simulink model "ACC_model"  (R2021a)
settings: Solver=VariableStepAuto  StartTime=0.0  StopTime=300  RelTol=1e-3
model workspace (MAT data in the model file):
  d0 = 0
undefined symbols (not defined in the file): sigbuilder_block
libraries: simulink x9, pid_lib x2
settings Model: Creator=david  LastModifiedBy=david
settings SolverCC: ZeroCrossAlgorithm=Adaptive
settings DebuggingCC: IgnoredZcDiagnostic=none

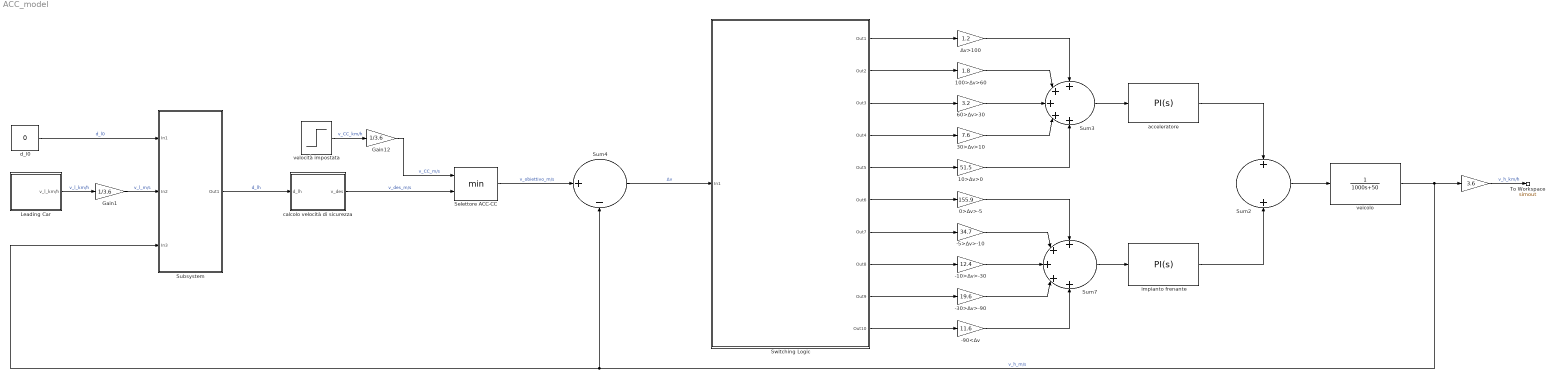
== system ACC_model ==
  " " : Gain  Gain=3.6
  -10>Δv>-30 : Gain  Gain=12.4
  -30>Δv>-90 : Gain  Gain=19.6
  -5>Δv>-10 : Gain  Gain=34.7
  -90<Δv : Gain  Gain=11.6
  0>Δv>-5 : Gain  Gain=155.9
  100>Δv>60 : Gain  Gain=1.8
  10>Δv>0 : Gain  Gain=51.5
  30>Δv>10 : Gain  Gain=7.6
  60>Δv>30 : Gain  Gain=3.2
  Gain1 : Gain  Gain=1/3.6
  Gain12 : Gain  Gain=1/3.6
  Leading Car : Subsystem  Tag=STV Subsys  LoadFcn=sigbuilder_block('load');  StartFcn=sigbuilder_block('start');  StopFcn=sigbuilder_block('stop');  ClipboardFcn=sigbuilder_block('clipboard');  mask(Sigbuilder block){tuvar=[0:10]}
      mask help: Simulink:masks:SigbuilderBlock_MD
      mask init:
      | if ~strcmp(get_param(bdroot(gcbh),'SimulationStatus'),'stopped') tuvar = sigbuilder_block('maskInit'); end
      settings: CopyFcn=sigbuilder_block('copy');  DeleteFcn=sigbuilder_block('delete');  ModelCloseFcn=sigbuilder_block('modelClose');  PreSaveFcn=sigbuilder_block('preSave');  PauseFcn=sigbuilder_block('pause');  ContinueFcn=sigbuilder_block('continue');  NameChangeFcn=sigbuilder_block('namechange');  OpenFcn=sigbuilder_block('open',[5.4 30 1525.2 738.6 ]);  CloseFcn=sigbuilder_block('close');
      mask Display: plot(0, 0, 100, 100,[2, 2, 32, 32, 2], [68, 8, 8, 68, 68],[32, 2], [38, 38], [32, 19, 2],[53, 60, 44], [32, 17, 17, 2],[16, 16, 31, 31]);txt = getActiveGroup(gcbh);text(2, 100, txt,'verticalAlignment', 'top');
  Selettore ACC-CC : MinMax  Inputs=2
  Subsystem : Subsystem
  Sum2 : Sum
  Sum3 : Sum  Inputs=+++++
  Sum4 : Sum  Inputs=|+-
  Sum7 : Sum  Inputs=+++++
  Switching Logic : Subsystem
  To Workspace : ToWorkspace  VariableName=simout  SaveFormat=Timeseries  SampleTime=-1
  acceleratore : pid_lib/PID Controller  Controller=PI  Form=Parallel  TimeDomain=Continuous-time  UseExternalTs=off  SampleTime=-1  IntegratorMethod=Forward Euler  FilterMethod=Forward Euler  ControllerParametersSource=internal  P=20  I=1  D=0  UseFilter=on  N=100  TunerSelectOption=Transfer Function Based (PID Tuner App)  InitialConditionSource=internal  InitialConditionForIntegrator=0  InitialConditionForFilter=0  DifferentiatorICPrevScaledInput=0  ExternalReset=none  TrackingMode=off  Kt=1  LimitOutput=off  SatLimitsSource=internal  UpperSaturationLimit=inf  LowerSaturationLimit=-inf  LinearizeAsGain=on  AntiWindupMode=none  Kb=1  POutMin=[]  POutMax=[]  IOutMin=[]  IOutMax=[]  DOutMin=[]  DOutMax=[]  NOutMin=[]  NOutMax=[]  SumOutMin=[]  SumOutMax=[]  SaturationOutMin=[]  SaturationOutMax=[]  PParamMin=[]  PParamMax=[]  IParamMin=[]  IParamMax=[]  DParamMin=[]  DParamMax=[]  NParamMin=[]  NParamMax=[]  KbParamMin=[]  KbParamMax=[]  KtParamMin=[]  KtParamMax=[]  KbOutMin=[]  KbOutMax=[]  KtOutMin=[]  KtOutMax=[]  IntegratorOutMin=[]  IntegratorOutMax=[]  FilterOutMin=[]  FilterOutMax=[]  SumI1OutMin=[]  SumI1OutMax=[]  SumI2OutMin=[]  SumI2OutMax=[]  SumI3OutMin=[]  SumI3OutMax=[]  SumI4OutMin=[]  SumI4OutMax=[]  SumDOutMin=[]  SumDOutMax=[]  DifferentiatorOutMin=[]  DifferentiatorOutMax=[]  FilterDiffOutCoefMin=[]  FilterDiffOutCoefMax=[]  ReciprocalOutMin=[]  ReciprocalOutMax=[]  SumDenOutMin=[]  SumDenOutMax=[]  SumNumOutMin=[]  SumNumOutMax=[]  DivideOutMin=[]  DivideOutMax=[]  UdiffTsProdOutMin=[]  UdiffTsProdOutMax=[]  NTsProdOutMin=[]  NTsProdOutMax=[]  UintegralTsProdOutMin=[]  UintegralTsProdOutMax=[]  UngainTsProdOutMin=[]  UngainTsProdOutMax=[]  IntegratorContinuousStateAttributes=''  IntegratorStateMustResolveToSignalObject=off  IntegratorRTWStateStorageClass=Auto  FilterContinuousStateAttributes=''  FilterStateMustResolveToSignalObject=off  FilterRTWStateStorageClass=Auto  ParallelPVariant=InternalParameters  IdealPVariant=Disabled  IVariant=InternalParameters  DVariant=Disabled  IntegratorVariant=Continuous  SatVariant=Disabled  AWVariant=Passthrough  PCopyVariant=Disabled  TRVariant=Disabled  FdbkBlocksVariant=Forward  IdealPFdbkVariant=Disabled  SatFdbkVariant=Disabled  DerivativeFilterVariant=Disabled  NVariant=Disabled  NCopyVariant=Disabled_SignalSpec  FilterICVariant=Disabled  IntegratorICVariant=InternalICs  ExternalResetVariant=Disabled  TRSumVariant=Passthrough  SumFdbkVariant=Disabled  SumVariant=Sum_PI  TsampFilterVariant=InternalTs  TsampNgainVariant=Passthrough  TsampIntegralVariant=Passthrough  ExternalSaturationOutDataTypeStr=Inherit: Same as second input
  calcolo velocità di sicurezza : MATLAB Function  TreatAsAtomicUnit=on
  d_l0 : Constant  Value=0
  impianto frenante : pid_lib/PID Controller  Controller=PI  Form=Parallel  TimeDomain=Continuous-time  UseExternalTs=off  SampleTime=-1  IntegratorMethod=Forward Euler  FilterMethod=Forward Euler  ControllerParametersSource=internal  P=20  I=1  D=0  UseFilter=on  N=100  TunerSelectOption=Transfer Function Based (PID Tuner App)  InitialConditionSource=internal  InitialConditionForIntegrator=0  InitialConditionForFilter=0  DifferentiatorICPrevScaledInput=0  ExternalReset=none  TrackingMode=off  Kt=1  LimitOutput=off  SatLimitsSource=internal  UpperSaturationLimit=inf  LowerSaturationLimit=-inf  LinearizeAsGain=on  AntiWindupMode=none  Kb=1  POutMin=[]  POutMax=[]  IOutMin=[]  IOutMax=[]  DOutMin=[]  DOutMax=[]  NOutMin=[]  NOutMax=[]  SumOutMin=[]  SumOutMax=[]  SaturationOutMin=[]  SaturationOutMax=[]  PParamMin=[]  PParamMax=[]  IParamMin=[]  IParamMax=[]  DParamMin=[]  DParamMax=[]  NParamMin=[]  NParamMax=[]  KbParamMin=[]  KbParamMax=[]  KtParamMin=[]  KtParamMax=[]  KbOutMin=[]  KbOutMax=[]  KtOutMin=[]  KtOutMax=[]  IntegratorOutMin=[]  IntegratorOutMax=[]  FilterOutMin=[]  FilterOutMax=[]  SumI1OutMin=[]  SumI1OutMax=[]  SumI2OutMin=[]  SumI2OutMax=[]  SumI3OutMin=[]  SumI3OutMax=[]  SumI4OutMin=[]  SumI4OutMax=[]  SumDOutMin=[]  SumDOutMax=[]  DifferentiatorOutMin=[]  DifferentiatorOutMax=[]  FilterDiffOutCoefMin=[]  FilterDiffOutCoefMax=[]  ReciprocalOutMin=[]  ReciprocalOutMax=[]  SumDenOutMin=[]  SumDenOutMax=[]  SumNumOutMin=[]  SumNumOutMax=[]  DivideOutMin=[]  DivideOutMax=[]  UdiffTsProdOutMin=[]  UdiffTsProdOutMax=[]  NTsProdOutMin=[]  NTsProdOutMax=[]  UintegralTsProdOutMin=[]  UintegralTsProdOutMax=[]  UngainTsProdOutMin=[]  UngainTsProdOutMax=[]  IntegratorContinuousStateAttributes=''  IntegratorStateMustResolveToSignalObject=off  IntegratorRTWStateStorageClass=Auto  FilterContinuousStateAttributes=''  FilterStateMustResolveToSignalObject=off  FilterRTWStateStorageClass=Auto  ParallelPVariant=InternalParameters  IdealPVariant=Disabled  IVariant=InternalParameters  DVariant=Disabled  IntegratorVariant=Continuous  SatVariant=Disabled  AWVariant=Passthrough  PCopyVariant=Disabled  TRVariant=Disabled  FdbkBlocksVariant=Forward  IdealPFdbkVariant=Disabled  SatFdbkVariant=Disabled  DerivativeFilterVariant=Disabled  NVariant=Disabled  NCopyVariant=Disabled_SignalSpec  FilterICVariant=Disabled  IntegratorICVariant=InternalICs  ExternalResetVariant=Disabled  TRSumVariant=Passthrough  SumFdbkVariant=Disabled  SumVariant=Sum_PI  TsampFilterVariant=InternalTs  TsampNgainVariant=Passthrough  TsampIntegralVariant=Passthrough  ExternalSaturationOutDataTypeStr=Inherit: Same as second input
  veicolo : TransferFcn  Denominator=[1000 50]
  velocità impostata : Step  After=70  SampleTime=0
  Δv>100 : Gain  Gain=1.2
  wires:
  calcolo velocità di sicurezza/1(v_des) -> Selettore ACC-CC/2  "v_des_m/s"
  velocità impostata/1 -> Gain12/1  "v_CC_km/h"
  Gain12/1 -> Selettore ACC-CC/1  "v_CC_m/s"
  -10>Δv>-30/1 -> Sum7/3
  Switching Logic/6(Out6) -> 0>Δv>-5/1
  Sum2/1 -> veicolo/1
  Switching Logic/7(Out7) -> -5>Δv>-10/1
  30>Δv>10/1 -> Sum3/4
  Switching Logic/3(Out3) -> 60>Δv>30/1
  Sum4/1 -> Switching Logic/1(In1)  "Δv"
  Δv>100/1 -> Sum3/1
  60>Δv>30/1 -> Sum3/3
  0>Δv>-5/1 -> Sum7/1
  -5>Δv>-10/1 -> Sum7/2
  Switching Logic/5(Out5) -> 10>Δv>0/1
  -30>Δv>-90/1 -> Sum7/4
  Switching Logic/10(Out10) -> -90<Δv/1
  Sum3/1 -> acceleratore/1
  Switching Logic/1(Out1) -> Δv>100/1
  -90<Δv/1 -> Sum7/5
  impianto frenante/1 -> Sum2/2
  Switching Logic/9(Out9) -> -30>Δv>-90/1
  Sum7/1 -> impianto frenante/1
  Switching Logic/8(Out8) -> -10>Δv>-30/1
  100>Δv>60/1 -> Sum3/2
  acceleratore/1 -> Sum2/1
  10>Δv>0/1 -> Sum3/5
  Switching Logic/4(Out4) -> 30>Δv>10/1
  Switching Logic/2(Out2) -> 100>Δv>60/1
  Selettore ACC-CC/1 -> Sum4/1  "v_obiettivo_m/s"
  veicolo/1 -> Subsystem/3(In3), Sum4/2, " "/1  "v_h_m/s"
  " "/1 -> To Workspace/1  "v_h_km/h"
  Leading Car/1(v_l_km/h) -> Gain1/1  "v_l_km/h"
  Gain1/1 -> Subsystem/2(In2)  "v_l_m/s"
  d_l0/1 -> Subsystem/1(In1)  "d_l0"
  Subsystem/1(Out1) -> calcolo velocità di sicurezza/1(d_lh)  "d_lh"

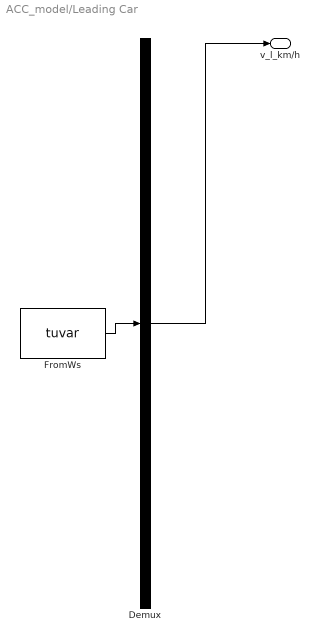
== system ACC_model/Leading Car ==
  Demux : Demux  Tag=STV Demux  Outputs=1
      settings: DisplayOption=none
  FromWs : FromWorkspace  Tag=STV FromWs  VariableName=tuvar
      SigBuilderData=|
      | common.afterFinalStr = 'Extrapolate'
      | common.sampleTime = 0
      | dataSet.timeRange = [0 300]
      | dataSet.name = ' '
      | sbobj.Groups.Name = ' '
      | sbobj.Groups.Signals.Name = 'v_l_km/h'
      | sbobj.Groups.Signals.XData = [0 110 110 300]
      | sbobj.Groups.Signals.YData = [70 70 0 0]
      | sbobj.Groups.TimeRange = [0 300]
  v_l_km/h : Outport  Tag=STV Outport
  wires:
  Demux/1 -> v_l_km/h/1
  FromWs/1 -> Demux/1

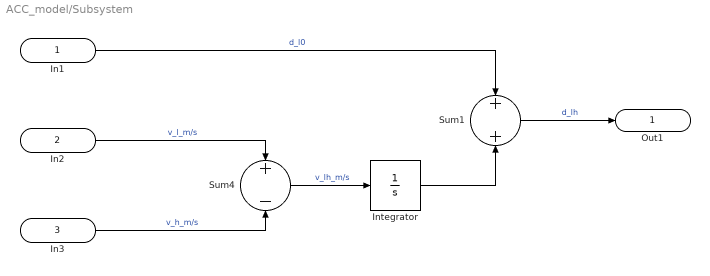
== system ACC_model/Subsystem ==
  In1 : Inport
  In2 : Inport  Port=2
  In3 : Inport  Port=3
  Integrator : Integrator
  Sum1 : Sum
  Sum4 : Sum  Inputs=+-
  Out1 : Outport
  wires:
  In1/1 -> Sum1/1  "d_l0"
  In2/1 -> Sum4/1  "v_l_m/s"
  In3/1 -> Sum4/2  "v_h_m/s"
  Sum4/1 -> Integrator/1  "v_lh_m/s"
  Integrator/1 -> Sum1/2
  Sum1/1 -> Out1/1  "d_lh"

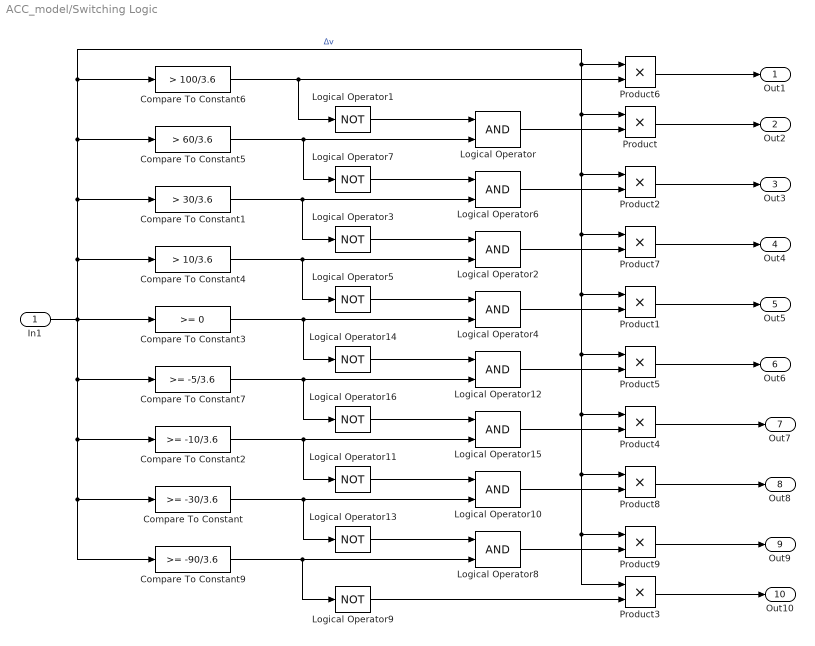
== system ACC_model/Switching Logic ==
  In1 : Inport
  Compare To Constant : simulink/Logic and Bit Operations/Compare To Constant  relop=>=  const=-30/3.6  OutDataTypeStr=boolean
  Compare To Constant1 : simulink/Logic and Bit Operations/Compare To Constant  relop=>  const=30/3.6  OutDataTypeStr=boolean
  Compare To Constant2 : simulink/Logic and Bit Operations/Compare To Constant  relop=>=  const=-10/3.6  OutDataTypeStr=boolean
  Compare To Constant3 : simulink/Logic and Bit Operations/Compare To Constant  relop=>=  const=0  OutDataTypeStr=boolean
  Compare To Constant4 : simulink/Logic and Bit Operations/Compare To Constant  relop=>  const=10/3.6  OutDataTypeStr=boolean
  Compare To Constant5 : simulink/Logic and Bit Operations/Compare To Constant  relop=>  const=60/3.6  OutDataTypeStr=boolean
  Compare To Constant6 : simulink/Logic and Bit Operations/Compare To Constant  relop=>  const=100/3.6  OutDataTypeStr=boolean
  Compare To Constant7 : simulink/Logic and Bit Operations/Compare To Constant  relop=>=  const=-5/3.6  OutDataTypeStr=boolean
  Compare To Constant9 : simulink/Logic and Bit Operations/Compare To Constant  relop=>=  const=-90/3.6  OutDataTypeStr=boolean
  Logical Operator{,2,4,6,8,10,12,15} (8 alike) : Logic  AllPortsSameDT=off  OutDataTypeStr=boolean
  Logical Operator{1,3,5,7,9,11,13..14,16} (9 alike) : Logic  Operator=NOT  AllPortsSameDT=off  OutDataTypeStr=boolean
  Product{,1..9} (10 alike) : Product
  Out1 : Outport
  Out2 : Outport  Port=2
  Out3 : Outport  Port=3
  Out4 : Outport  Port=4
  Out5 : Outport  Port=5
  Out6 : Outport  Port=6
  Out7 : Outport  Port=7
  Out8 : Outport  Port=8
  Out9 : Outport  Port=9
  Out10 : Outport  Port=10
  wires:
  Compare To Constant1/1 -> Logical Operator3/1, Logical Operator6/2
  Logical Operator6/1 -> Product2/2
  Compare To Constant3/1 -> Logical Operator14/1, Logical Operator4/2
  Logical Operator1/1 -> Logical Operator/1
  Product2/1 -> Out3/1
  Product6/1 -> Out1/1
  Logical Operator/1 -> Product/2
  Compare To Constant5/1 -> Logical Operator7/1, Logical Operator/2
  Product1/1 -> Out5/1
  Logical Operator7/1 -> Logical Operator6/1
  Logical Operator2/1 -> Product7/2
  Compare To Constant4/1 -> Logical Operator5/1, Logical Operator2/2
  Logical Operator4/1 -> Product1/2
  Logical Operator3/1 -> Logical Operator2/1
  Logical Operator5/1 -> Logical Operator4/1
  Compare To Constant6/1 -> Product6/2, Logical Operator1/1
  Product/1 -> Out2/1
  Product7/1 -> Out4/1
  Logical Operator9/1 -> Product3/2
  Logical Operator10/1 -> Product8/2
  Product5/1 -> Out6/1
  Product4/1 -> Out7/1
  Logical Operator13/1 -> Logical Operator8/1
  Compare To Constant9/1 -> Logical Operator9/1, Logical Operator8/2
  Logical Operator15/1 -> Product4/2
  Product3/1 -> Out10/1
  Logical Operator16/1 -> Logical Operator15/1
  Product9/1 -> Out9/1
  Logical Operator8/1 -> Product9/2
  In1/1 -> Compare To Constant5/1, Compare To Constant6/1, Product/1, Product2/1, Product7/1, Product3/1, Product9/1, Product8/1, Product4/1, Product5/1, Product1/1, Product6/1, Compare To Constant1/1, Compare To Constant4/1, Compare To Constant9/1, Compare To Constant/1, Compare To Constant2/1, Compare To Constant7/1, Compare To Constant3/1  "Δv"
  Logical Operator12/1 -> Product5/2
  Compare To Constant/1 -> Logical Operator13/1, Logical Operator10/2
  Logical Operator14/1 -> Logical Operator12/1
  Logical Operator11/1 -> Logical Operator10/1
  Compare To Constant7/1 -> Logical Operator16/1, Logical Operator12/2
  Compare To Constant2/1 -> Logical Operator11/1, Logical Operator15/2
  Product8/1 -> Out8/1

== matlab function ACC_model/calcolo velocità di sicurezza ==
  data: v_des output; d_lh input
function v_des = fcn(d_lh)
h_1=1.511;   %definizione h_1
h_2=0.088;   %definizione h_2
d_f= 2.25;   %definizione d_f
if (d_lh<d_f)
    v_des=0;    
else
    v_des = (-h_1+sqrt(h_1^2-4*h_2*(d_f-d_lh)))/(2*h_2);
end
